simulink model "WaterRunner"  (Simulink 8.1)
settings: Solver=ode15s  StartTime=0.0  StopTime=10  FixedStep=1e-3  RelTol=1e-3
values from neighbouring files (symbols this model uses):
  frame_inertia = diag([Ix,Iy,Iz])    [simParams.m]
  frame_mass = .140-4*motor_mass    (= 0.1)    [simParams.m]
  L2_inertia = diag([I 0 I])    [simParams.m]
  L2_mass = CF_density*cross_area*L2    (= 0.0002653496)    [simParams.m]
  L3_inertia = diag([I 0 I])    [simParams.m]
  L3_mass = CF_density*cross_area*L3    (= 0.0009104656)    [simParams.m]
  L4_inertia = diag([I 0 I])    [simParams.m]
  L4_mass = CF_density*cross_area*L4    (= 0.0005696496)    [simParams.m]
  water_level = 0    [simParams.m]
undefined symbols (not defined in the file): initRobHeight
libraries: mblibv1 x18, WaterRunner_lib x14, simulink x1
settings Model: Creator=fumiyaiida  LastModifiedBy=nitisht  SimulationMode=accelerator
settings SolverCC: ZeroCrossControl=DisableAll
settings OptimizationCC: InitFltsAndDblsToZero=on  EfficientMapNaN2IntZero=off  SimCompilerOptimization=On
settings DebuggingCC: SaveWithParameterizedLinksMsg=none  SignalResolutionControl=TryResolveAllWithWarning  SolverPrmCheckMsg=none  MultiTaskDSMMsg=warning  MultiTaskCondExecSysMsg=none  StrictBusMsg=None
settings HardwareCC: ProdBitPerLong=64  ProdBitPerPointer=64  ProdIntDivRoundTo=Zero  ProdEndianess=LittleEndian  ProdWordSize=64  ProdHWDeviceType=Intel->x86-64  TargetBitPerLong=64  TargetBitPerPointer=64  TargetIntDivRoundTo=Zero  TargetEndianess=LittleEndian  TargetWordSize=64  TargetHWDeviceType=MATLAB Host  ProdEqTarget=off
settings RTWCC: RTWCompilerOptimization=On
settings CodeAppCC: MaxIdLength=128
settings SimMechanicsCC: WarnOnSingularInitialAssembly=on  VisSampleTime=0.001  AnimationDelay=1  LastVizWinPosition=[2 523 1918 455]  CamPosition=[0.788259;0.0309166;13.4817;]  CamTarget=[0.742597;-0.00982635;-0.00911848;]  CamUpVector=[-0.000894773;0.999995;-0.00301701;]  CamHeight=2.55  VisBackgroundColor=[0.9;0.9;0.95;]  DefaultBodyColor=[1;0;0;]
settings ConfigurationSet: Description=SimMechanics 2G

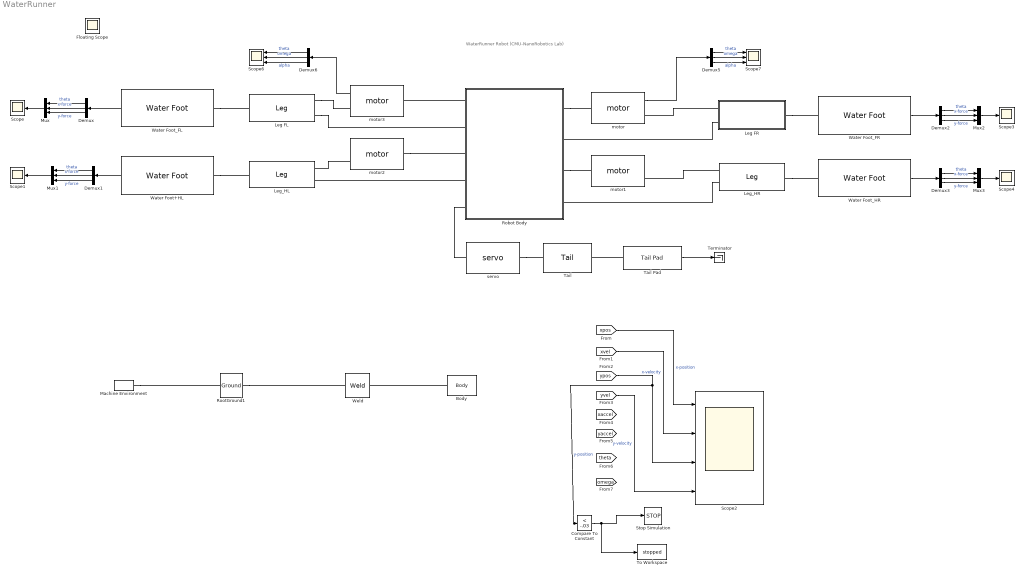
== system WaterRunner ==
  note: WaterRunner Robot
      | (CMU-NanoRobotics Lab)
  Body : mblibv1/Bodies/Body  LConnTagsString=CG  UpdateFromCAD=off  DialogClass=MechanicalBodyBlock  Mass=1  MassUnits=kg  InertiaUnits=kg*m^2  Inertia=eye(3)  Shape=Cylinder  ShapeDims=[1 1]  ShapeUnits=m  ShapeUse=false  Density=1  DensityUnits=kg/m^3  DensityUse=false  GraphicsMode=CONVHULL  BodyColorSelMode=COLORPALETTE  BodyColor=[0.83137 0.81569 0.78431]  AttachedToCS=CG  CG=Left$CG$[0 0 0]$WORLD$WORLD$m$[0 0 0]$Euler X-Y-Z$deg$WORLD$true$none  WorkingFrames=Left$CS1$[-0.5 water_level -0.2 ]$CG$CG$m$[0 0 0]$Euler X-Y-Z$deg$WORLD$false$none#Left$CS2$[-0.5 water_level 0.2 ]$CG$CG$m$[0 0 0]$Euler X-Y-Z$deg$WORLD$false$none#Left$CS3$[4 water_level -0.2 ]$CG$CG$m$[0 0 0]$Euler X-Y-Z$deg$WORLD$false$none#Left$CS4$[4 water_level 0.2 ]$CG$CG$m$[0 0 0]$Euler X-Y-Z$deg$WORLD$false$none  CGPos=[0 0 0]  CGRot=[0 0 0]  CS0Pos=[]  CS0Rot=[]  CS1Pos=[-0.5 water_level -0.2 ]  CS1Rot=[0 0 0]  CS2Pos=[-0.5 water_level 0.2 ]  CS2Rot=[0 0 0]  CS3Pos=[4 water_level -0.2 ]  CS3Rot=[0 0 0]  CS4Pos=[4 water_level 0.2 ]  CS4Rot=[0 0 0]  CS5Pos=[]  CS5Rot=[]  CS6Pos=[]  CS6Rot=[]  CS7Pos=[]  CS7Rot=[]  CS8Pos=[]  CS8Rot=[]  CS9Pos=[]  CS9Rot=[]  CS10Pos=[]  CS10Rot=[]  CS11Pos=[]  CS11Rot=[]  CS12Pos=[]  CS12Rot=[]  CS13Pos=[]  CS13Rot=[]  CS14Pos=[]  CS14Rot=[]  CS15Pos=[]  CS15Rot=[]  CS16Pos=[]  CS16Rot=[]  CS17Pos=[]  CS17Rot=[]  CS18Pos=[]  CS18Rot=[]  CS19Pos=[]  CS19Rot=[]  CS20Pos=[]  CS20Rot=[]
  Compare To Constant : simulink/Logic and Bit Operations/Compare To Constant  relop=<  const=-.03  OutDataTypeStr=boolean
  Demux{,1..3,5..6} (6 alike) : Demux  Outputs=3
  Leg FL : WaterRunner_lib/Leg
  Leg FR : Subsystem  AncestorBlock=WaterRunner_lib/Leg
      mask help: mask for leg
  Leg_HL : WaterRunner_lib/Leg
  Leg_HR : WaterRunner_lib/Leg
  Machine Environment : mblibv1/Bodies/Machine Environment  PortType=env  PhysicalDomain=Mechanical  DialogTemplateClass=MECH.MachineEnvironment  SyncWhenCopied=off  Gravity=[0 -9.81 0]  GravityUnits=m/s^2  GravityAsSignal=off  Dimensionality=Auto-detect  AnalysisType=Forward dynamics  LinearAssemblyTolerance=1e-3  LinearAssemblyToleranceUnits=m  AngularAssemblyTolerance=1e-3  AngularAssemblyToleranceUnits=rad  ConstraintSolverType=Stabilizing  ConstraintRelTolerance=1e-4  ConstraintAbsTolerance=1e-4  UseRobustSingularityHandling=off  RedundancyAnalysisToleranceType=Automatically select tolerance  RedundancyAnalysisTolerance=1e-14  StatePerturbationType=Fixed  PerturbationSize=1e-5  VisualizeMachine=on  BodyVisualizationType=Use model default body geometries  BodyColorSelMode=Use model default  DefaultBodyColor=[1 0 0]
  Mux{,1..3} (4 alike) : Mux  Inputs=3
  Robot Body : Subsystem  AncestorBlock=WaterRunner_lib/Robot Body  mask{initRobHeight=initRobHeight}
      mask prompts: initRobHeight "height"
  RootGround1 : mblibv1/Bodies/Ground  UpdateFromCAD=on  LeftPortType=env  RightPortType=workingframe  PhysicalDomain=Mechanical  DialogClass=GroundBlock  CoordPosition=[0 0 0]  CoordPositionUnits=m  StateVectorMgrId=-1  MachineId=[0 0]  ShowEnvPort=on
  Scope{,1,3..4} (4 alike) : Scope
      Scope settings: ShowLegends=on  TimeRange=2  YMin=-2.5  YMax=2  SaveName=FootForce_FL
      Scope1 settings: ShowLegends=on  TimeRange=2  YMin=-2.5  YMax=2  SaveName=FootForce_HL
      Scope3 settings: ShowLegends=on  TimeRange=2  YMin=-2.5  YMax=2  SaveName=FootForce_FR
      Scope4 settings: ShowLegends=on  TimeRange=2  YMin=-2.5  YMax=2  SaveName=FootForce_HR
  Scope2 : Scope  NumInputPorts=4
      settings: ShowLegends=on  TimeRange=10  YMin=-0.5~0~-0.005~-0.2  YMax=3~2.5~0.035~0.4  SaveName=position
  Scope6 : Scope  NumInputPorts=3
      settings: TimeRange=2  YMin=-20~-90~-50000  YMax=-2.5~0~30000  SaveName=MotorMotion1
  Scope7 : Scope  NumInputPorts=3
      settings: TimeRange=2  YMin=-17.5~-90~-70000  YMax=0~0~30000  SaveName=MotorMotion
  Stop Simulation : Stop
  Tail : WaterRunner_lib/Tail
  Tail Pad : WaterRunner_lib/Tail Pad
  Terminator : Terminator
  To Workspace : ToWorkspace  VariableName=stopped  SampleTime=-1  SaveFormat=Timeseries
  Water Foot+HL : WaterRunner_lib/Water Foot
  Water Foot_FL : WaterRunner_lib/Water Foot
  Water Foot_FR : WaterRunner_lib/Water Foot
  Water Foot_HR : WaterRunner_lib/Water Foot
  Weld : mblibv1/Joints/Weld  LConnTagsString=__newl0  RConnTagsString=__newr0  UpdateFromCAD=off  NumSAPorts=0  CutJoint=off  MarkAsCut=off  Primitives=weld  PrimitiveProps=W$WORLD$[0 0 0]$weld  DialogClass=JointBlock  WAxis=[0 0 0]
  motor : WaterRunner_lib/motor  variableName=work_FR  ic_angle=0
  motor1 : WaterRunner_lib/motor  variableName=work_HR  ic_angle=pi
  motor2 : WaterRunner_lib/motor  variableName=work_HL  ic_angle=0
  motor3 : WaterRunner_lib/motor  variableName=work_FL  ic_angle=pi
  servo : WaterRunner_lib/servo  tail_angle=tail_angle  VariableName=work_tail
  Floating Scope : Scope
      settings: Floating=on
  wires:
  Water Foot_FL/1 -> Demux/1
  Demux/1 -> Mux/1  "theta"
  Demux/2 -> Mux/2  "x-force"
  Demux/3 -> Mux/3  "y-force"
  Mux/1 -> Scope/1
  [ypos] -> Scope2/3, Compare To Constant/1  "y-position"
  Water Foot+HL/1 -> Demux1/1
  Demux1/1 -> Mux1/1  "theta"
  Demux1/2 -> Mux1/2  "x-force"
  Demux1/3 -> Mux1/3  "y-force"
  Mux1/1 -> Scope1/1
  Mux2/1 -> Scope3/1
  Demux2/3 -> Mux2/3  "y-force"
  Demux2/2 -> Mux2/2  "x-force"
  Demux2/1 -> Mux2/1  "theta"
  Water Foot_FR/1 -> Demux2/1
  Mux3/1 -> Scope4/1
  Demux3/3 -> Mux3/3  "y-force"
  Demux3/2 -> Mux3/2  "x-force"
  Demux3/1 -> Mux3/1  "theta"
  Water Foot_HR/1 -> Demux3/1
  Compare To Constant/1 -> Stop Simulation/1, To Workspace/1
  Demux5/3 -> Scope7/3  "alpha"
  Demux5/2 -> Scope7/2  "omega"
  Demux5/1 -> Scope7/1  "theta"
  motor/1 -> Demux5/1
  Demux6/3 -> Scope6/3  "alpha"
  Demux6/2 -> Scope6/2  "omega"
  Demux6/1 -> Scope6/1  "theta"
  motor3/1 -> Demux6/1
  Tail Pad/1 -> Terminator/1
  [xpos] -> Scope2/1  "x-position"
  [xvel] -> Scope2/2  "x-velocity"
  [yvel] -> Scope2/4  "y-velocity"
  connections:
  RootGround1/RConn1 -- Weld/LConn1
  Body/LConn1 -- Weld/RConn1
  Robot Body/RConn1 -- motor/LConn1
  Leg FR/LConn2 -- Robot Body/RConn2
  Leg FR/LConn1 -- motor/RConn1
  Robot Body/RConn3 -- motor1/LConn1
  Leg_HR/LConn1 -- motor1/RConn1
  Leg_HR/LConn2 -- Robot Body/RConn4
  Water Foot+HL/LConn1 -- Leg_HL/RConn1
  Water Foot_FL/LConn1 -- Leg FL/RConn1
  Robot Body/LConn4 -- Leg_HL/LConn2
  Leg FR/RConn1 -- Water Foot_FR/LConn1
  Leg_HR/RConn1 -- Water Foot_HR/LConn1
  Robot Body/LConn1 -- motor3/LConn1
  motor2/RConn1 -- Leg_HL/LConn1
  motor2/LConn1 -- Robot Body/LConn3
  Leg FL/LConn2 -- Robot Body/LConn2
  Machine Environment/RConn1 -- RootGround1/LConn1
  Leg FL/LConn1 -- motor3/RConn1
  Robot Body/LConn5 -- servo/LConn1
  servo/RConn1 -- Tail/LConn1
  Tail Pad/LConn1 -- Tail/RConn1

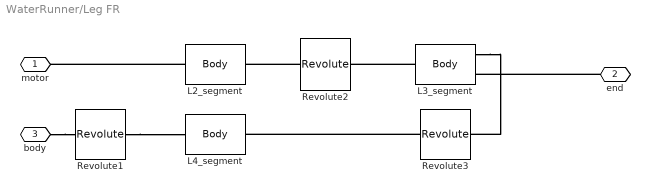
== system WaterRunner/Leg FR ==
  L2_segment : mblibv1/Bodies/Body  LConnTagsString=CS1  RConnTagsString=CS2  UpdateFromCAD=off  DialogClass=MechanicalBodyBlock  Mass=L2_mass  MassUnits=kg  InertiaUnits=kg*m^2  Inertia=L2_inertia  Shape=Cylinder  ShapeDims=[1 1]  ShapeUnits=m  ShapeUse=false  Density=1  DensityUnits=kg/m^3  DensityUse=false  GraphicsMode=CONVHULL  BodyColorSelMode=COLORPALETTE  BodyColor=[0 0 0]  AttachedToCS=CG  CG=Left$CG$L2_CG$CS1$CS1$m$[0 0 0]$Euler X-Y-Z$deg$WORLD$false$none  WorkingFrames=Left$CS1$L2_CS1$Adjoining$Adjoining$m$[0 0 0]$Euler X-Y-Z$deg$WORLD$true$none#Right$CS2$L2_CS2$CS1$CS1$m$[0 0 0]$Euler X-Y-Z$deg$WORLD$true$none  CGPos=L2_CG  CGRot=[0 0 0]  CS0Pos=[]  CS0Rot=[]  CS1Pos=L2_CS1  CS1Rot=[0 0 0]  CS2Pos=L2_CS2  CS2Rot=[0 0 0]  CS3Pos=[]  CS3Rot=[]  CS4Pos=[]  CS4Rot=[]  CS5Pos=[]  CS5Rot=[]  CS6Pos=[]  CS6Rot=[]  CS7Pos=[]  CS7Rot=[]  CS8Pos=[]  CS8Rot=[]  CS9Pos=[]  CS9Rot=[]  CS10Pos=[]  CS10Rot=[]  CS11Pos=[]  CS11Rot=[]  CS12Pos=[]  CS12Rot=[]  CS13Pos=[]  CS13Rot=[]  CS14Pos=[]  CS14Rot=[]  CS15Pos=[]  CS15Rot=[]  CS16Pos=[]  CS16Rot=[]  CS17Pos=[]  CS17Rot=[]  CS18Pos=[]  CS18Rot=[]  CS19Pos=[]  CS19Rot=[]  CS20Pos=[]  CS20Rot=[]
  L3_segment : mblibv1/Bodies/Body  LConnTagsString=CS1  RConnTagsString=CS2|CS3  UpdateFromCAD=off  DialogClass=MechanicalBodyBlock  Mass=L3_mass  MassUnits=kg  InertiaUnits=kg*m^2  Inertia=L3_inertia  Shape=Cylinder  ShapeDims=[1 1]  ShapeUnits=m  ShapeUse=false  Density=1  DensityUnits=kg/m^3  DensityUse=false  GraphicsMode=CONVHULL  BodyColorSelMode=COLORPALETTE  BodyColor=[0 0 0]  AttachedToCS=CG  CG=Left$CG$L3_CG$CS1$CS1$m$[0 0 0]$Euler X-Y-Z$rad$CS1$false$none  WorkingFrames=Left$CS1$L3_CS1$Adjoining$Adjoining$m$L3_ori$Euler X-Y-Z$rad$Adjoining$true$none#Right$CS2$L3_CS2$CS1$CS1$m$[0 0 0]$Euler X-Y-Z$rad$CS1$true$none#Right$CS3$L3_CS3$CS1$CS1$m$[0 0 0]$Euler X-Y-Z$rad$CS1$true$none  CGPos=L3_CG  CGRot=[0 0 0]  CS0Pos=[]  CS0Rot=[]  CS1Pos=L3_CS1  CS1Rot=L3_ori  CS2Pos=L3_CS2  CS2Rot=[0 0 0]  CS3Pos=L3_CS3  CS3Rot=[0 0 0]  CS4Pos=[]  CS4Rot=[]  CS5Pos=[]  CS5Rot=[]  CS6Pos=[]  CS6Rot=[]  CS7Pos=[]  CS7Rot=[]  CS8Pos=[]  CS8Rot=[]  CS9Pos=[]  CS9Rot=[]  CS10Pos=[]  CS10Rot=[]  CS11Pos=[]  CS11Rot=[]  CS12Pos=[]  CS12Rot=[]  CS13Pos=[]  CS13Rot=[]  CS14Pos=[]  CS14Rot=[]  CS15Pos=[]  CS15Rot=[]  CS16Pos=[]  CS16Rot=[]  CS17Pos=[]  CS17Rot=[]  CS18Pos=[]  CS18Rot=[]  CS19Pos=[]  CS19Rot=[]  CS20Pos=[]  CS20Rot=[]
  L4_segment : mblibv1/Bodies/Body  LConnTagsString=CS1  RConnTagsString=CS2  UpdateFromCAD=off  DialogClass=MechanicalBodyBlock  Mass=L4_mass  MassUnits=kg  InertiaUnits=kg*m^2  Inertia=L4_inertia  Shape=Cylinder  ShapeDims=[1 1]  ShapeUnits=m  ShapeUse=false  Density=1  DensityUnits=kg/m^3  DensityUse=false  GraphicsMode=CONVHULL  BodyColorSelMode=COLORPALETTE  BodyColor=[0 0 0]  AttachedToCS=CG  CG=Left$CG$L4_CG$CS1$CS1$m$[0 0 0]$Euler X-Y-Z$rad$CS1$false$none  WorkingFrames=Left$CS1$L4_CS1$Adjoining$Adjoining$m$L4_ori$Euler X-Y-Z$rad$Adjoining$true$none#Right$CS2$L4_CS2$CS1$CS1$m$[0 0 0]$Euler X-Y-Z$rad$CS1$true$none  CGPos=L4_CG  CGRot=[0 0 0]  CS0Pos=[]  CS0Rot=[]  CS1Pos=L4_CS1  CS1Rot=L4_ori  CS2Pos=L4_CS2  CS2Rot=[0 0 0]  CS3Pos=[]  CS3Rot=[]  CS4Pos=[]  CS4Rot=[]  CS5Pos=[]  CS5Rot=[]  CS6Pos=[]  CS6Rot=[]  CS7Pos=[]  CS7Rot=[]  CS8Pos=[]  CS8Rot=[]  CS9Pos=[]  CS9Rot=[]  CS10Pos=[]  CS10Rot=[]  CS11Pos=[]  CS11Rot=[]  CS12Pos=[]  CS12Rot=[]  CS13Pos=[]  CS13Rot=[]  CS14Pos=[]  CS14Rot=[]  CS15Pos=[]  CS15Rot=[]  CS16Pos=[]  CS16Rot=[]  CS17Pos=[]  CS17Rot=[]  CS18Pos=[]  CS18Rot=[]  CS19Pos=[]  CS19Rot=[]  CS20Pos=[]  CS20Rot=[]
  Revolute1 : mblibv1/Joints/Revolute  LConnTagsString=__newl0  RConnTagsString=__newr0  UpdateFromCAD=off  NumSAPorts=0  CutJoint=off  MarkAsCut=off  Primitives=prismatic  PrimitiveProps=R1$World$[0 0 1]$revolute  DialogClass=JointBlock  R1Axis=[0 0 1]
  Revolute2 : mblibv1/Joints/Revolute  LConnTagsString=__newl0  RConnTagsString=__newr0  UpdateFromCAD=off  NumSAPorts=0  CutJoint=on  MarkAsCut=off  Primitives=prismatic  PrimitiveProps=R1$World$[0 0 1]$revolute  DialogClass=JointBlock  R1Axis=[0 0 1]
  Revolute3 : mblibv1/Joints/Revolute  LConnTagsString=__newl0  RConnTagsString=__newr0  UpdateFromCAD=off  NumSAPorts=0  CutJoint=off  MarkAsCut=off  Primitives=prismatic  PrimitiveProps=R1$World$[0 0 1]$revolute  DialogClass=JointBlock  R1Axis=[0 0 1]
  motor : PMIOPort  Port=1  Side=Left
  end : PMIOPort  Port=2  Side=Right
  body : PMIOPort  Port=3  Side=Left
  connections:
  L2_segment/LConn1 -- motor/RConn1
  Revolute2/LConn1 -- L2_segment/RConn1
  L3_segment/LConn1 -- Revolute2/RConn1
  L3_segment/RConn1 -- Revolute3/RConn1
  Revolute1/RConn1 -- L4_segment/LConn1
  Revolute3/LConn1 -- L4_segment/RConn1
  body/RConn1 -- Revolute1/LConn1
  end/RConn1 -- L3_segment/RConn2

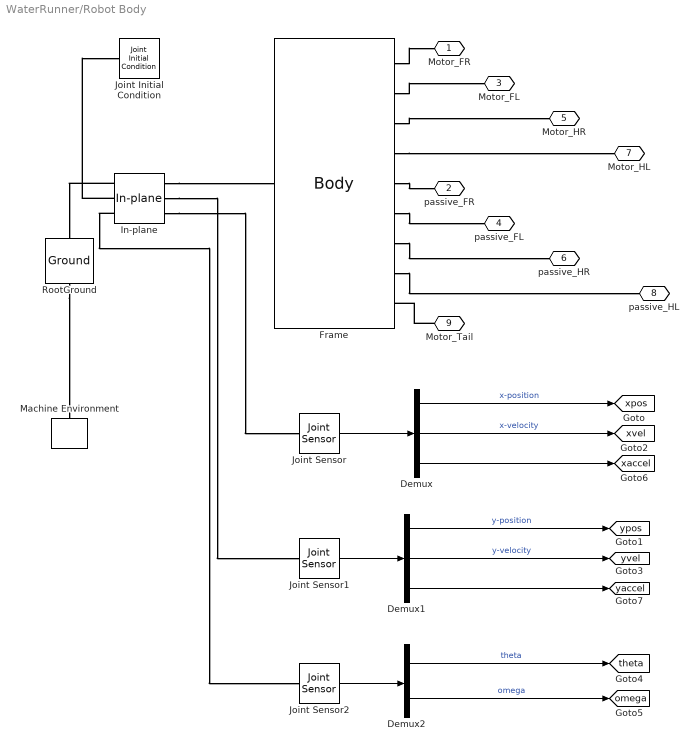
== system WaterRunner/Robot Body ==
  Demux : Demux  Outputs=3
  Demux1 : Demux  Outputs=3
  Demux2 : Demux  Outputs=2
  Frame : mblibv1/Bodies/Body  LConnTagsString=CS1  RConnTagsString=CS6|CS7|CS8|CS9|CS10|CS11|CS12|CS13|CS14  UpdateFromCAD=off  DialogClass=MechanicalBodyBlock  Mass=frame_mass  MassUnits=kg  InertiaUnits=kg*m^2  Inertia=frame_inertia  Shape=Cylinder  ShapeDims=[1 1]  ShapeUnits=m  ShapeUse=false  Density=1  DensityUnits=kg/m^3  DensityUse=false  GraphicsMode=CONVHULL  BodyColorSelMode=COLORPALETTE  BodyColor=[0 0 1]  AttachedToCS=CG  CG=Left$CG$frame_CG$WORLD$WORLD$m$[0 0 0]$Euler X-Y-Z$deg$WORLD$false$none  WorkingFrames=Left$CS1$frame_CA$World$World$m$[0 0 0]$Euler X-Y-Z$deg$WORLD$true$none#Right$CS2$frame_FR$World$World$m$[0 0 0]$Euler X-Y-Z$deg$WORLD$false$none#Right$CS4$frame_FL$World$World$m$[0 0 0]$Euler X-Y-Z$deg$WORLD$false$none#Right$CS3$frame_HR$World$World$m$[0 0 0]$Euler X-Y-Z$deg$WORLD$false$none#Right$CS5$frame_HL$WORLD$WORLD$m$[0 0 0]$Euler X-Y-Z$deg$WORLD$false$none#Right$CS6$frame_motor_FR$WORLD$WORLD$m$[0 0 0]$Euler X-Y-Z$deg$WORLD$true$none#Right$CS7$frame_motor_FL$WORLD$WORLD$m$[0 0 0]$Euler X-Y-Z$deg$WORLD$true$none#Right$CS8$frame_motor_HR$WORLD$WORLD$m$[0 0 0]$Euler X-Y-Z$deg$WORLD$true$none#Right$CS9$frame_motor_HL$WORLD$WORLD$m$[0 0 0]$Euler X-Y-Z$deg$WORLD$true$none#Right$CS10$frame_passive_FR$WORLD$WORLD$m$[0 0 0]$Euler X-Y-Z$deg$WORLD$true$none#Right$CS11$frame_passive_FL$WORLD$WORLD$m$[0 0 0]$Euler X-Y-Z$deg$WORLD$true$none#Right$CS12$frame_passive_HR$WORLD$WORLD$m$[0 0 0]$Euler X-Y-Z$deg$WORLD$true$none#Right$CS13$frame_passive_HL$WORLD$WORLD$m$[0 0 0]$Euler X-Y-Z$deg$WORLD$true$none#Right$CS14$frame_motor_Tail$WORLD$WORLD$m$[0 0 0]$Euler X-Y-Z$deg$WORLD$true$none  CGPos=frame_CG  CGRot=[0 0 0]  CS0Pos=[]  CS0Rot=[]  CS1Pos=frame_CA  CS1Rot=[0 0 0]  CS2Pos=frame_FR  CS2Rot=[0 0 0]  CS3Pos=frame_HR  CS3Rot=[0 0 0]  CS4Pos=frame_FL  CS4Rot=[0 0 0]  CS5Pos=frame_HL  CS5Rot=[0 0 0]  CS6Pos=frame_motor_FR  CS6Rot=[0 0 0]  CS7Pos=frame_motor_FL  CS7Rot=[0 0 0]  CS8Pos=frame_motor_HR  CS8Rot=[0 0 0]  CS9Pos=frame_motor_HL  CS9Rot=[0 0 0]  CS10Pos=frame_passive_FR  CS10Rot=[0 0 0]  CS11Pos=frame_passive_FL  CS11Rot=[0 0 0]  CS12Pos=frame_passive_HR  CS12Rot=[0 0 0]  CS13Pos=frame_passive_HL  CS13Rot=[0 0 0]  CS14Pos=frame_motor_Tail  CS14Rot=[0 0 0]  CS15Pos=[]  CS15Rot=[]  CS16Pos=[]  CS16Rot=[]  CS17Pos=[]  CS17Rot=[]  CS18Pos=[]  CS18Rot=[]  CS19Pos=[]  CS19Rot=[]  CS20Pos=[]  CS20Rot=[]
  In-plane : mblibv1/Joints/In-plane  LConnTagsString=__newl0|SA1|SA2  RConnTagsString=__newr0|SA1|SA2  UpdateFromCAD=off  NumSAPorts=4  CutJoint=off  MarkAsCut=off  Primitives=prismatic  PrimitiveProps=P1$World$[1 0 0]$prismatic#P2$World$[0 1 0]$prismatic  DialogClass=JointBlock  P1Axis=[1 0 0]  P2Axis=[0 1 0]
  Joint Initial Condition : mblibv1/Sensors &  Actuators/Joint Initial Condition  UpdateFromCAD=off  LeftPortType=blob  RightPortType=blob  PhysicalDomain=mechanical  DialogClass=InitialConditionBlock  InitialConditions=P1$true$0$m$deg$0$m/s$deg/s#P2$false$initRobHeight$m$deg$0$m/s$deg/s#P3$false$0$m$deg$0$m/s$deg/s#R1$false$0$m$rad$0$m/s$rad/s#R2$false$0$m$deg$0$m/s$deg/s#R3$false$0$m$deg$0$m/s$deg/s#S$false$0$m$deg$0$m/s$deg/s  P1PIC=0  P1VIC=0  P2PIC=0  P2VIC=0  P3PIC=0  P3VIC=0  R1PIC=0  R1VIC=0  R2PIC=0  R2VIC=0  R3PIC=0  R3VIC=0  SPIC=0  SVIC=0
  Joint Sensor : mblibv1/Sensors &  Actuators/Joint Sensor  UpdateFromCAD=off  PhysicalDomain=Mechanical  PortType=blob  Muxed=on  Pose=off  Angle=on  AngleUnits=deg  ArcVelocity=off  ArcVelocityUnits=deg/s  ArcAcceleration=off  ArcAccelerationUnits=deg/s^2  CoordPosition=on  CoordPositionUnits=m  Velocity=on  VelocityUnits=m/s  Acceleration=on  AccelerationUnits=m/s^2  Quaternion=on  QuaternionDT=off  QuaternionDDT=off  QuaternionUnits=off  OutputVector=[1]  ActiveIO=on  Width=3  DialogClass=MechanicalSensorBlock  Primitive=P1  Force=off  ForceUnits=N  Torque=off  TorqueUnits=N*m  ReferenceFrame=Absolute (World)  ReactionSensedSide=Base  ReactionReferenceFrame=Absolute (World)  ReactionForce=off  ReactionForceUnits=N  ReactionMoment=off  ReactionMomentUnits=N*m
  Joint Sensor1 : mblibv1/Sensors &  Actuators/Joint Sensor  UpdateFromCAD=off  PhysicalDomain=Mechanical  PortType=blob  Muxed=on  Pose=off  Angle=on  AngleUnits=deg  ArcVelocity=off  ArcVelocityUnits=deg/s  ArcAcceleration=off  ArcAccelerationUnits=deg/s^2  CoordPosition=on  CoordPositionUnits=m  Velocity=on  VelocityUnits=m/s  Acceleration=on  AccelerationUnits=m/s^2  Quaternion=on  QuaternionDT=off  QuaternionDDT=off  QuaternionUnits=off  OutputVector=[1]  ActiveIO=on  Width=3  DialogClass=MechanicalSensorBlock  Primitive=P2  Force=off  ForceUnits=N  Torque=off  TorqueUnits=N*m  ReferenceFrame=Absolute (World)  ReactionSensedSide=Base  ReactionReferenceFrame=Absolute (World)  ReactionForce=off  ReactionForceUnits=N  ReactionMoment=off  ReactionMomentUnits=N*m
  Joint Sensor2 : mblibv1/Sensors &  Actuators/Joint Sensor  UpdateFromCAD=off  PhysicalDomain=Mechanical  PortType=blob  Muxed=on  Pose=off  Angle=on  AngleUnits=rad  ArcVelocity=on  ArcVelocityUnits=rad/s  ArcAcceleration=off  ArcAccelerationUnits=deg/s^2  CoordPosition=on  CoordPositionUnits=m  Velocity=on  VelocityUnits=m/s  Acceleration=off  AccelerationUnits=m/s^2  Quaternion=on  QuaternionDT=off  QuaternionDDT=off  QuaternionUnits=off  OutputVector=[1]  ActiveIO=on  Width=2  DialogClass=MechanicalSensorBlock  Primitive=P1  Force=off  ForceUnits=N  Torque=off  TorqueUnits=N*m  ReferenceFrame=Absolute (World)  ReactionSensedSide=Base  ReactionReferenceFrame=Absolute (World)  ReactionForce=off  ReactionForceUnits=N  ReactionMoment=off  ReactionMomentUnits=N*m
  Machine Environment : mblibv1/Bodies/Machine Environment  PortType=env  PhysicalDomain=Mechanical  DialogTemplateClass=MECH.MachineEnvironment  SyncWhenCopied=off  Gravity=[0 -9.81 0]  GravityUnits=m/s^2  GravityAsSignal=off  Dimensionality=Auto-detect  AnalysisType=Forward dynamics  LinearAssemblyTolerance=1e-3  LinearAssemblyToleranceUnits=m  AngularAssemblyTolerance=1e-3  AngularAssemblyToleranceUnits=rad  ConstraintSolverType=Stabilizing  ConstraintRelTolerance=1e-4  ConstraintAbsTolerance=1e-4  UseRobustSingularityHandling=off  RedundancyAnalysisToleranceType=Automatically select tolerance  RedundancyAnalysisTolerance=1e-14  StatePerturbationType=Fixed  PerturbationSize=1e-5  VisualizeMachine=on  BodyVisualizationType=Use model default body geometries  BodyColorSelMode=Use model default  DefaultBodyColor=[1 0 0]
  RootGround : mblibv1/Bodies/Ground  UpdateFromCAD=on  LeftPortType=env  RightPortType=workingframe  PhysicalDomain=Mechanical  DialogClass=GroundBlock  CoordPosition=[0 0 0]  CoordPositionUnits=m  StateVectorMgrId=-1  MachineId=[0 0]  ShowEnvPort=on
  Motor_FR : PMIOPort  Port=1  Side=Right
  passive_FR : PMIOPort  Port=2  Side=Right
  Motor_FL : PMIOPort  Port=3  Side=Left
  passive_FL : PMIOPort  Port=4  Side=Left
  Motor_HR : PMIOPort  Port=5  Side=Right
  passive_HR : PMIOPort  Port=6  Side=Right
  Motor_HL : PMIOPort  Port=7  Side=Left
  passive_HL : PMIOPort  Port=8  Side=Left
  Motor_Tail : PMIOPort  Port=9  Side=Left
  tag scope: omega=global, theta=global, xaccel=global, xpos=global, xvel=global, yaccel=global, ypos=global, yvel=global
  wires:
  Demux1/3 -> [yaccel]
  Demux/3 -> [xaccel]
  Joint Sensor2/1 -> Demux2/1
  Demux2/2 -> [omega]  "omega"
  Demux2/1 -> [theta]  "theta"
  Demux1/2 -> [yvel]  "y-velocity"
  Demux1/1 -> [ypos]  "y-position"
  Demux/2 -> [xvel]  "x-velocity"
  Demux/1 -> [xpos]  "x-position"
  Joint Sensor1/1 -> Demux1/1
  Joint Sensor/1 -> Demux/1
  connections:
  In-plane/LConn3 -- Joint Sensor2/LConn1
  In-plane/RConn3 -- Joint Sensor/LConn1
  Motor_Tail/RConn1 -- Frame/RConn9
  In-plane/RConn2 -- Joint Sensor1/LConn1
  In-plane/LConn2 -- Joint Initial Condition/RConn1
  Frame/RConn8 -- passive_HL/RConn1
  Frame/RConn7 -- passive_HR/RConn1
  Frame/RConn6 -- passive_FL/RConn1
  Frame/RConn5 -- passive_FR/RConn1
  Frame/RConn4 -- Motor_HL/RConn1
  Frame/RConn3 -- Motor_HR/RConn1
  Frame/RConn2 -- Motor_FL/RConn1
  Frame/RConn1 -- Motor_FR/RConn1
  In-plane/LConn1 -- RootGround/RConn1
  RootGround/LConn1 -- Machine Environment/RConn1
  In-plane/RConn1 -- Frame/LConn1
